simulink model "System_Model"  (R2022b)
settings: Solver=VariableStepAuto  StartTime=0.0  StopTime=10.0  RelTol=1e-3
values from neighbouring files (symbols this model uses):
  S = [m , I_y, Damping_matrix(1,1), Damping_matrix(2,2), Damping_matrix(3,3)]    [Inizializzazione.m]
settings Model: Creator=angel  LastModifiedBy=anton
settings ModelReferenceCC: EnableRefExpFcnMdlSchedulingChecks=on

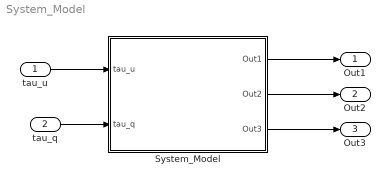
== system System_Model ==
  tau_u : Inport
  tau_q : Inport  Port=2
  System_Model : Subsystem
  Out1 : Outport
  Out2 : Outport  Port=2
  Out3 : Outport  Port=3
  wires:
  tau_u/1 -> System_Model/1(tau_u)
  tau_q/1 -> System_Model/2(tau_q)
  System_Model/1(Out1) -> Out1/1
  System_Model/2(Out2) -> Out2/1
  System_Model/3(Out3) -> Out3/1

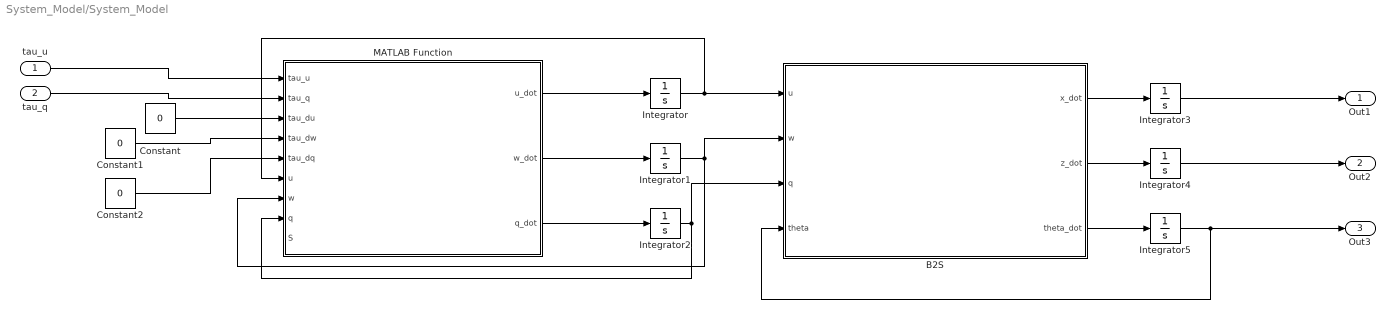
== system System_Model/System_Model ==
  tau_u : Inport
  tau_q : Inport  Port=2
  B2S : MATLAB Function  TreatAsAtomicUnit=on
  Constant : Constant  Value=0
  Constant1 : Constant  Value=0
  Constant2 : Constant  Value=0
  Integrator{,1..5} (6 alike) : Integrator
  MATLAB Function : MATLAB Function  TreatAsAtomicUnit=on  mask{M=S}
      mask prompts: M "Costanti del sistema"
  Out1 : Outport
  Out2 : Outport  Port=2
  Out3 : Outport  Port=3
  wires:
  B2S/1(x_dot) -> Integrator3/1
  B2S/3(theta_dot) -> Integrator5/1
  tau_q/1 -> MATLAB Function/2(tau_q)
  tau_u/1 -> MATLAB Function/1(tau_u)
  Integrator4/1 -> Out2/1
  Constant1/1 -> MATLAB Function/4(tau_dw)
  B2S/2(z_dot) -> Integrator4/1
  MATLAB Function/2(w_dot) -> Integrator1/1
  MATLAB Function/3(q_dot) -> Integrator2/1
  Integrator2/1 -> B2S/3(q), MATLAB Function/8(q)
  Integrator5/1 -> Out3/1, B2S/4(theta)
  Integrator1/1 -> MATLAB Function/7(w), B2S/2(w)
  MATLAB Function/1(u_dot) -> Integrator/1
  Constant/1 -> MATLAB Function/3(tau_du)
  Integrator3/1 -> Out1/1
  Constant2/1 -> MATLAB Function/5(tau_dq)
  Integrator/1 -> B2S/1(u), MATLAB Function/6(u)

== matlab function System_Model/B2S ==
  data: u input; x_dot output; w input; q input; theta input; z_dot output; theta_dot output
function [x_dot, z_dot, theta_dot] = BodyToSpatial(u, w, q, theta)

R = [cos(theta) sin(theta) 0; -sin(theta) cos(theta) 0; 0 0 1];   % matrice di rotazione B2S

[x_dot, z_dot, theta_dot]' = R*[u w q]';

== matlab function System_Model/MATLAB Function ==
  data: tau_u input; tau_q input; tau_du input; tau_dw input; tau_dq input; u input; u_dot output; w input; q input; w_dot output; q_dot output; S input
function [u_dot, w_dot, q_dot] = BodyDynamics(tau_u, tau_q, tau_du, tau_dw, tau_dq,u, w, q, S)

[m , lx, lz, I_y, C_lu,C_lw,C_qq,C_qu,C_qw,C_lq] = S;
B=[m 0 0; 0 m 0; 0 0 I]; %Matrice di massa
C=[C_lu+C_qu*abs(u) 0 m*w;
   0 C_lw+C_qw*abs(w) -m*u ;
   -m*w m*u C_lq+C_qq*abs(q)]; %Matrice dei termini di Coriolis
Tau=[tau_u;0; tau_q];
Tau_d=[tau_du; tau_dw; tau_dq];
S_Body=[u;w;q];
S_Body_dot =inv(B)*(Tau+Tau_d-C*S_Body);
u_dot = S_Body_dot(1);
w_dot = S_Body_dot(2);
q_dot = S_Body_dot(3);
